simulink model "final_sim"  (R2019b)
settings: Solver=VariableStepAuto  StartTime=0.0  StopTime=10.0  RelTol=1e-3
settings Model: Creator=Mertcan  LastModifiedBy=Mertcan

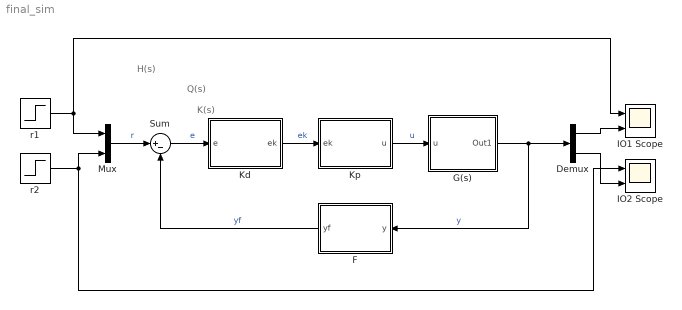
== system final_sim ==
  note: H(s)
  note: Q(s)
  note: K(s)
  Demux : Demux  Outputs=2
  F : MATLAB Function  TreatAsAtomicUnit=on
  G(s) : Subsystem
  IO1 Scope : Scope  NumInputPorts=2
  IO2 Scope : Scope  NumInputPorts=2
  Kd : MATLAB Function  TreatAsAtomicUnit=on
  Kp : MATLAB Function  TreatAsAtomicUnit=on
  Mux : Mux  Inputs=2
  Sum : Sum  Inputs=|+-
  r1 : Step  SampleTime=0
  r2 : Step  SampleTime=0
  wires:
  Kd/1(ek) -> Kp/1(ek)  "ek"
  Sum/1 -> Kd/1(e)  "e"
  Mux/1 -> Sum/1  "r"
  r1/1 -> IO1 Scope/1, Mux/1
  r2/1 -> Mux/2, IO2 Scope/1
  F/1(yf) -> Sum/2  "yf"
  Kp/1(u) -> G(s)/1(u)  "u"
  G(s)/1(Out1) -> Demux/1, F/1(y)  "y"
  Demux/1 -> IO1 Scope/2
  Demux/2 -> IO2 Scope/2

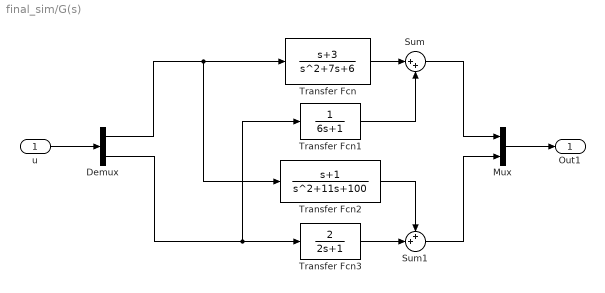
== system final_sim/G(s) ==
  u : Inport
  Demux : Demux  Outputs=2
  Mux : Mux  Inputs=2
  Sum : Sum  Inputs=|++
  Sum1 : Sum  Inputs=++|
  Transfer Fcn : TransferFcn  Numerator=[1 3]  Denominator=[1 7 6]
  Transfer Fcn1 : TransferFcn  Denominator=[6 1]
  Transfer Fcn2 : TransferFcn  Numerator=[1 1]  Denominator=[1 11 100]
  Transfer Fcn3 : TransferFcn  Numerator=[2]  Denominator=[2 1]
  Out1 : Outport
  wires:
  u/1 -> Demux/1
  Transfer Fcn/1 -> Sum/1
  Mux/1 -> Out1/1
  Transfer Fcn1/1 -> Sum/2
  Transfer Fcn2/1 -> Sum1/1
  Transfer Fcn3/1 -> Sum1/2
  Sum1/1 -> Mux/2
  Sum/1 -> Mux/1
  Demux/1 -> Transfer Fcn2/1, Transfer Fcn/1
  Demux/2 -> Transfer Fcn1/1, Transfer Fcn3/1

== matlab function final_sim/Kp ==
  data: ek input; u output
function u = Kp(ek)

K = [2.0202, -1.0101
    -0.010101, 0.505051];

u = K*ek;

== matlab function final_sim/Kd ==
  data: e input; ek output
function ek = k1k2(e)

k1 = 30;
k2 = 30;

K = [k1 0
     0 k2];

ek = K*e;

== matlab function final_sim/F ==
  data: y input; yf output
function yf = I(y)

F = eye(2);

yf = F*y;
